simulink model "lqg_cartpend_sim_modified4"  (R2015a)
settings: Solver=ode45  StartTime=0.0  StopTime=10  RelTol=1e-3
InitFcn:
  | 'simulink_cartPend_initialize.m'
values from neighbouring files (symbols this model uses):
  b = pendPar.b    [cartPendMatrix.m]    (also in cartPendVector.m = par.b; run_cartPend.m = 1; run_cartPend_LQG.m = 1; run_cartPend_LQR.m = 1)
  g = pendPar.g    [cartPendMatrix.m]    (also in cartPendVector.m = par.g; run_cartPend.m = -10; run_cartPend_LQG.m = -10; run_cartPend_LQR.m = -10)
  K = place(A, B, p )    [run_cartPend.m]    (also in run_cartPend_LQG.m = [0,0,0,0]; run_cartPend_LQR.m = lqr( A,B,Q,R); run_cartPend_linearizedControl.m; simulink_cartPend_initialize.m = [0,0,0,0])
  L = pendPar.L    [cartPendMatrix.m]    (also in run_cartPend.m = 2; run_cartPend_LQG.m = 2; run_cartPend_LQR.m = 2; run_cartPend_kalmanFilter.m = 2)
  mc = pendPar.mc    [cartPendMatrix.m]    (also in cartPendVector.m = par.mc; run_cartPend.m = 5; run_cartPend_LQG.m = 5; run_cartPend_LQR.m = 5)
  mp = pendPar.mp    [cartPendMatrix.m]    (also in cartPendVector.m = par.mp; run_cartPend.m = 1; run_cartPend_LQG.m = 1; run_cartPend_LQR.m = 1)
  y0 = [-4,0,pi*10/12,0]    [run_cartPend.m]    (also in run_cartPend_LQG.m = [-4,0,pi*9/12,0]; run_cartPend_LQR.m = [-4,0,pi*9/12,0]; run_cartPend_kalmanFilter.m = [-4,0,pi*9/12,0]; run_cartPend_linearizedControl.m)
settings Model: Creator=Thomas  LastModifiedBy=Thomas
settings DataIOCC: InitialState=yIn

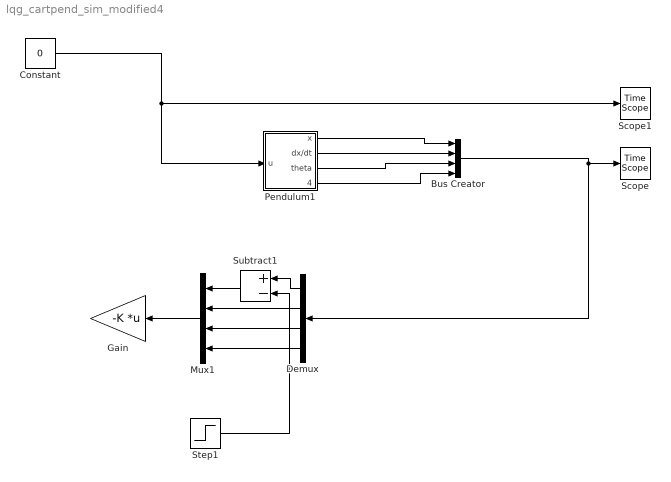
== system lqg_cartpend_sim_modified4 ==
  Bus Creator : BusCreator
  Constant : Constant  Value=0
  Demux : Demux
  Gain : Gain  Gain=-K  Multiplication=Matrix(K*u) (u vector)
  Mux1 : Mux
  Pendulum1 : Subsystem  mask(Inverted pendulum on cart){mc=mc, mp=mp, L=L, g=g, b=b}
      mask prompts: mc "Mass of cart (kg):"; mp "Mass of pendulum (kg):"; L "Distance to pendulum center of mass(m):"; g "Acceleration of gravity (m/s^2):"; b "Damping of cart (kg/s)"
      mask help: Unmask and double-click to see dynamics
      mask Help: Nonlinear dynamics of inverted pendulum on cart.
  Scope : TimeScope
  Scope1 : TimeScope
  Step1 : Step  Time=10  After=0  SampleTime=0
  Subtract1 : Sum  Inputs=+-
  wires:
  Demux/2 -> Mux1/2
  Demux/4 -> Mux1/4
  Demux/3 -> Mux1/3
  Mux1/1 -> Gain/1
  Subtract1/1 -> Mux1/1
  Demux/1 -> Subtract1/1
  Step1/1 -> Subtract1/2
  Bus Creator/1 -> Demux/1, Scope/1
  Pendulum1/4(d theta/dt) -> Bus Creator/4
  Pendulum1/3("theta ") -> Bus Creator/3
  Pendulum1/2(dx/dt) -> Bus Creator/2
  Pendulum1/1(x) -> Bus Creator/1
  Constant/1 -> Scope1/1, Pendulum1/1(u)

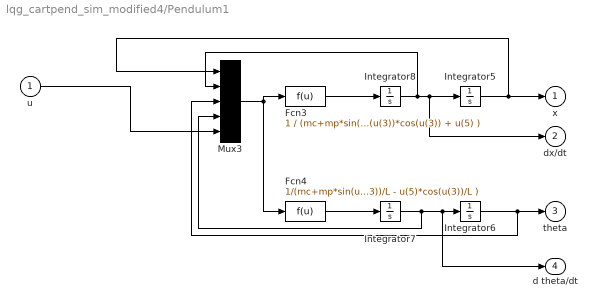
== system lqg_cartpend_sim_modified4/Pendulum1 ==
  u : Inport
  Fcn3 : Fcn  Expr="1 / (mc+mp*sin(u(3))^2)  * ( -u(2)*b +u(4)^2*mp*L*sin(u(3)) - mp*g*sin(u(3))*cos(u(3)) + u(5) )"
  Fcn4 : Fcn  Expr=1/(mc+mp*sin(u(3))^2)*( u(2)*b*cos(u(3))/L - sin(u(4))^2*mp*sin(u(3))*cos(u(3)) + (mc+mp)*g*sin(u(3))/L - u(5)*cos(u(3))/L )
  Integrator5 : Integrator  InitialCondition=y0(1)  ContinuousStateAttributes='x'
  Integrator6 : Integrator  InitialCondition=y0(3)  ContinuousStateAttributes='theta'
  Integrator7 : Integrator  InitialCondition=y0(4)  ContinuousStateAttributes='theta_dot'
  Integrator8 : Integrator  InitialCondition=y0(2)  ContinuousStateAttributes='xDot'
  Mux3 : Mux  Inputs=5
  x : Outport  InitialOutput=0
  dx/dt : Outport  Port=2  InitialOutput=0
  "theta " : Outport  Port=3  InitialOutput=0
  d theta/dt : Outport  Port=4  InitialOutput=0
  wires:
  Integrator5/1 -> Mux3/1, x/1
  Fcn4/1 -> Integrator7/1
  Mux3/1 -> Fcn4/1, Fcn3/1
  Fcn3/1 -> Integrator8/1
  Integrator8/1 -> Mux3/2, dx/dt/1, Integrator5/1
  Integrator7/1 -> Mux3/4, d theta/dt/1, Integrator6/1
  Integrator6/1 -> Mux3/3, "theta "/1
  u/1 -> Mux3/5
